simulink model "HomeExperiment"  (R2022b)
settings: Solver=FixedStepAuto  StartTime=0.0  StopTime=inf  RelTol=1e-3  EnableMultiTasking=on
model workspace (MAT data in the model file):
  sampleTime = 0.01
libraries: arduinolib x6
settings Model: FPTRunName=Active  ExtModeTrigDuration=2  Creator=The MathWorks, Inc.  LastModifiedBy=arkad
settings SolverCC: AlgebraicLoopSolver=TrustRegion
settings DataIOCC: LimitDataPoints=on  ReturnWorkspaceOutputs=off
settings OptimizationCC: ExpressionDepthLimit=2147483647  LifeSpan=Inf  MaxStackSize=64
settings DebuggingCC: UnderspecifiedInitializationDetection=Classic  MergeDetectMultiDrivingBlocksExec=none  ParameterOverflowMsg=none  ParameterUnderflowMsg=error  ParameterPrecisionLossMsg=none  FcnCallInpInsideContextMsg=warning  UnconnectedInputMsg=warning  UnconnectedOutputMsg=warning  UnconnectedLineMsg=warning  AllowSymbolicDim=off  StateNameClashWarn=warning  SFUnexpectedBacktrackingDiag=warning  SFNoUnconditionalDefaultTransitionDiag=warning  SFExecutionAtInitializationDiag=none  SFMachineParentedDataDiag=warning  ArithmeticOperatorsInVariantConditions=warning
settings HardwareCC: ProdBitPerInt=16  ProdBitPerPointer=16  ProdBitPerSizeT=16  ProdBitPerPtrDiffT=16  ProdLargestAtomicFloat=None  ProdWordSize=8  ProdHWDeviceType=Atmel->AVR
settings ModelReferenceCC: EnableRefExpFcnMdlSchedulingChecks=on  PropagateSignalLabelsOutOfModel=off
settings SFSimCC: SimUseLocalCustomCode=off  MATLABDynamicMemAlloc=off
settings RTWCC: Description=Embedded Coder  SystemTargetFile=ert.tlc  HardwareBoard=Arduino Uno  TemplateMakefile=ert_default_tmf  GenerateReport=on  RTWVerbose=off  RTWUseLocalCustomCode=off  Toolchain=Arduino AVR  BuildConfiguration=Faster Runs  LaunchReport=on  DLArmComputeVersion=19.05
settings CodeAppCC: ForceParamTrailComments=on  OperatorAnnotations=on  StateflowObjectComments=on  MATLABSourceComments=on
settings ERTTargetCC: MultiwordLength=2048  ERTCustomFileBanners=off  SupportContinuousTime=on  SupportNonInlinedSFcns=on  RemoveResetFunc=off  SupportVariableSizeSignals=on  ModelStepFunctionPrototypeControlCompliant=off  ExtModeTransport=3  ExtModeStaticAlloc=on  ExtModeAutomaticAllocSize=off  ExtModeStaticAllocSize=250  ExtModeMexFile=ext_xcp  ExtModeIntrfLevel=Level2 - Open
settings ConfigComp: CovMetricSettings=dw  CovSaveCumulativeToWorkspaceVar=on  CovSaveSingleToWorkspaceVar=on  CovExternalEMLEnable=off  CovSFcnEnable=off

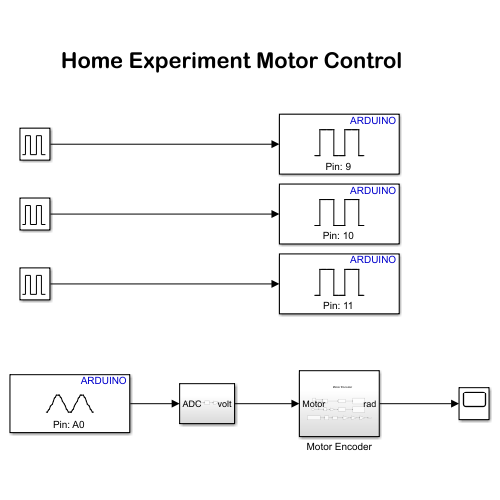
[thumbnail: Simulink's stored preview of the top-level diagram]
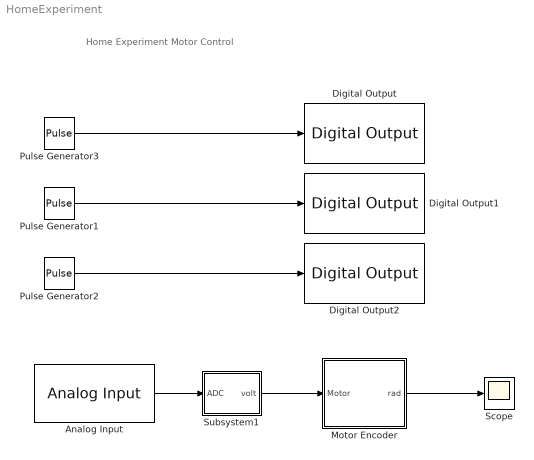
== system HomeExperiment ==
  note: Home Experiment Motor Control
  Analog Input : arduinolib/Analog Input  pinNumber=0  ReadResultsOnly=off  ConversionTriggerSource=Software  ExternalTriggerType=uint32( 0 )  OutputDataType=uint16  EnableConversionCompleteNotify=off  EnableOuputStatus=off  SampleTime=sampleTime  blockPlatform=arduino
  Digital Output : arduinolib/Digital Output  pinNumber=9  Direction=output  blockPlatform=arduino
  Digital Output1 : arduinolib/Digital Output  pinNumber=10  Direction=output  blockPlatform=arduino
  Digital Output2 : arduinolib/Digital Output  pinNumber=11  Direction=output  blockPlatform=arduino
  Motor Encoder : Subsystem
  Pulse Generator1 : DiscretePulseGenerator  PulseType=Time based  PulseWidth=50  SampleTime=sampleTime
  Pulse Generator2 : DiscretePulseGenerator  PulseType=Time based  Period=5  PulseWidth=50  SampleTime=sampleTime
  Pulse Generator3 : DiscretePulseGenerator  PulseType=Time based  Period=1  PulseWidth=50  SampleTime=sampleTime
  Scope : Scope
  Subsystem1 : Subsystem
  wires:
  Pulse Generator3/1 -> Digital Output/1
  Pulse Generator1/1 -> Digital Output1/1
  Pulse Generator2/1 -> Digital Output2/1
  Motor Encoder/1(rad) -> Scope/1
  Analog Input/1 -> Subsystem1/1(ADC)
  Subsystem1/1(volt) -> Motor Encoder/1(Motor)

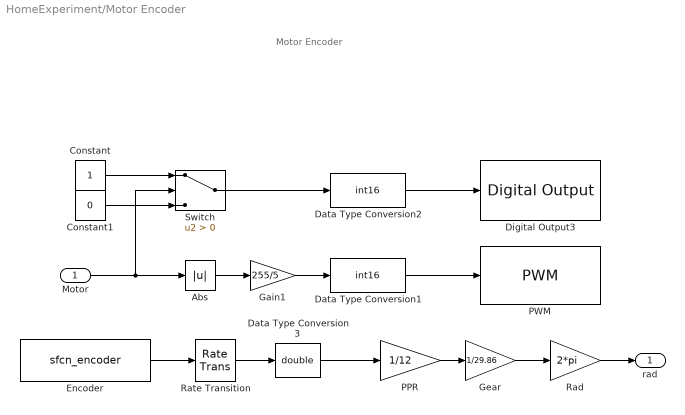
== system HomeExperiment/Motor Encoder ==
  note: Motor Encoder
  Motor : Inport
  Abs : Abs  SaturateOnIntegerOverflow=off
  Constant : Constant  SampleTime=sampleTime
  Constant1 : Constant  Value=0  SampleTime=sampleTime
  Data Type Conversion1 : DataTypeConversion  OutDataTypeStr=int16  SaturateOnIntegerOverflow=off  RndMeth=Floor
  Data Type Conversion2 : DataTypeConversion  OutDataTypeStr=int16  SaturateOnIntegerOverflow=off  RndMeth=Floor
  Data Type Conversion3 : DataTypeConversion  OutDataTypeStr=double  SaturateOnIntegerOverflow=off  RndMeth=Floor
  Digital Output3 : arduinolib/Digital Output  pinNumber=4  Direction=output  blockPlatform=arduino
  Encoder : S-Function  InitFcn=try, set_param(gcb,'FunctionName','sfcn_encoder'), end  FunctionName=sfcn_encoder  Parameters=uint8(0),uint8(2),uint8(3)  SFunctionModules=sfcn_encoder_wrapper  SFunctionDeploymentMode=off  EnableBusSupport=off  mask(S-Function Builder){}
      mask init:
      | val = [[.9  0.75 0.75 1 1 .9 .9 1]',[1 1 0.75 0.75 .9 .9 1 .9]'];try , sys = get_param(gcb,'SfunBuilderFcnName');if isempty(sys), sys = get_param(gcb,'FunctionName'); end,catch, sys = get_param(gcb,'FunctionName'); end
      settings: CopyFcn=set_param(gcbh,'LinkStatus','none')  PreSaveFcn=try, set_param(gcb,'FunctionName','sfcn_encoder'), end  OpenFcn=sfunctionwizard(gcbh)
      mask Display: plot(val(:,1),val(:,2)),disp(sys), port_label('output',1,'pos')
  Gain1 : Gain  Gain=255/5
  Gear : Gain  Gain=1/29.86
  PPR : Gain  Gain=1/12
  PWM : arduinolib/PWM  pinNumber=5  frequencyType=Default  desiredFrequency=490.2  achievableFrequency=490.2
  Rad : Gain  Gain=2*pi
  Rate Transition : RateTransition  OutPortSampleTime=sampleTime
  Switch : Switch  Criteria=u2 > Threshold  SaturateOnIntegerOverflow=off  InputSameDT=off
  rad : Outport
  wires:
  Data Type Conversion2/1 -> Digital Output3/1
  Switch/1 -> Data Type Conversion2/1
  Motor/1 -> Switch/2, Abs/1
  Constant1/1 -> Switch/3
  Constant/1 -> Switch/1
  Gain1/1 -> Data Type Conversion1/1
  Abs/1 -> Gain1/1
  Data Type Conversion1/1 -> PWM/1
  Rad/1 -> rad/1
  PPR/1 -> Gear/1
  Gear/1 -> Rad/1
  Data Type Conversion3/1 -> PPR/1
  Rate Transition/1 -> Data Type Conversion3/1
  Encoder/1 -> Rate Transition/1

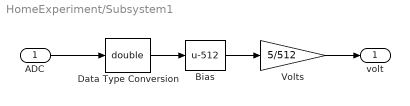
== system HomeExperiment/Subsystem1 ==
  ADC : Inport
  Bias : Bias  Bias=-512  SaturateOnIntegerOverflow=off
  Data Type Conversion : DataTypeConversion  OutDataTypeStr=double  SaturateOnIntegerOverflow=off  RndMeth=Floor
  Volts : Gain  Gain=5/512
  volt : Outport
  wires:
  Volts/1 -> volt/1
  Data Type Conversion/1 -> Bias/1
  Bias/1 -> Volts/1
  ADC/1 -> Data Type Conversion/1
